simulink model "pid_18a"  (R2018a)
settings: Solver=FixedStepDiscrete  StartTime=0.0  StopTime=10.0  FixedStep=0.1  RelTol=1e-3
undefined symbols (not defined in the file or in its folder): DiscIntNeverNeededParam
settings Model: Creator=kika  LastModifiedBy=kika
settings DataIOCC: ReturnWorkspaceOutputs=on
settings SFSimCC: SimUseLocalCustomCode=on
settings RTWCC: RTWUseLocalCustomCode=on

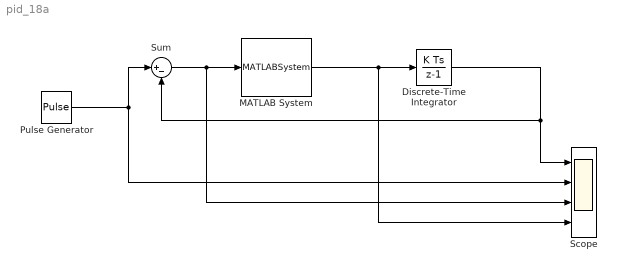
== system pid_18a ==
  Discrete-Time Integrator : DiscreteIntegrator  SampleTime=-1  ICPrevOutput=DiscIntNeverNeededParam  ICPrevScaledInput=DiscIntNeverNeededParam
  MATLAB System : MATLABSystem  System=PID  kp=2  ki=0  kd=0  dt=0.05  kt=1  u_max=1  u_min=-1  SimulateUsing=Interpreted execution
      mask Type: PID
      mask Display:
      | disp('PID');
      | port_label('input',1,'e');
      | port_label('output',1,'y');
  Pulse Generator : DiscretePulseGenerator  PulseType=Time based  Period=5  PulseWidth=50
  Scope : Scope  NumInputPorts=4
  Sum : Sum  Inputs=|+-
  wires:
  MATLAB System/1 -> Scope/4, Discrete-Time Integrator/1
  Sum/1 -> Scope/3, MATLAB System/1
  Pulse Generator/1 -> Sum/1, Scope/2
  Discrete-Time Integrator/1 -> Sum/2, Scope/1
